simulink model "aeb"  (R2024a)
settings: Solver=VariableStepAuto  StartTime=0.0  StopTime=10.0  RelTol=1e-3
libraries: raspberrypisensorlib x1, autosarlibaprouting x1, raspberrypiNetworklib x1
settings Model: Creator=dahyun  LastModifiedBy=dahyun

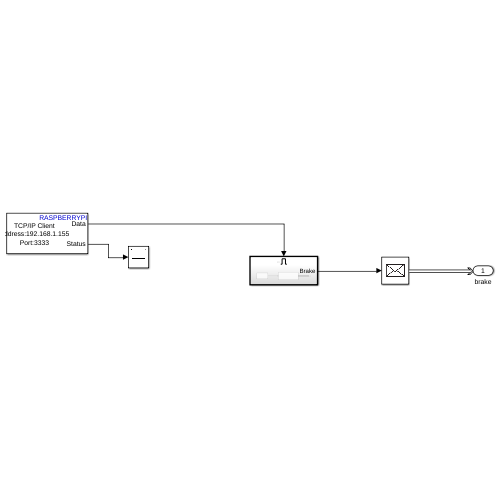
[thumbnail: Simulink's stored preview of the top-level diagram]
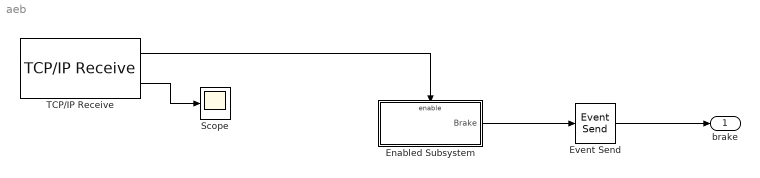
== system aeb ==
  Enabled Subsystem : Subsystem  TreatAsAtomicUnit=on
  Event Send : autosarlibaprouting/Event Send
  Scope : Scope
  TCP/IP Receive : raspberrypiNetworklib/TCP//IP Receive  Mode_=Client  LocalServerPort_=25000  RemoteAddr_=192.168.1.155  RemoteServerPort_=3333  DataType_=uint8  DataSize_=1  SampleTime_=0.1  SimulateUsing=Code generation  ClientPortBindingSelection_=off  ClientPortToBind_=35000  BlockingMode_=off  BlockTimeout_=0.1  BlockPlatform=RASPBERRYPI
  brake : Outport  InputPortMessageModes=m
  wires:
  Enabled Subsystem/1(Brake) -> Event Send/1
  TCP/IP Receive/2 -> Scope/1
  TCP/IP Receive/1 -> Enabled Subsystem/Enable
  Event Send/1 -> brake/1

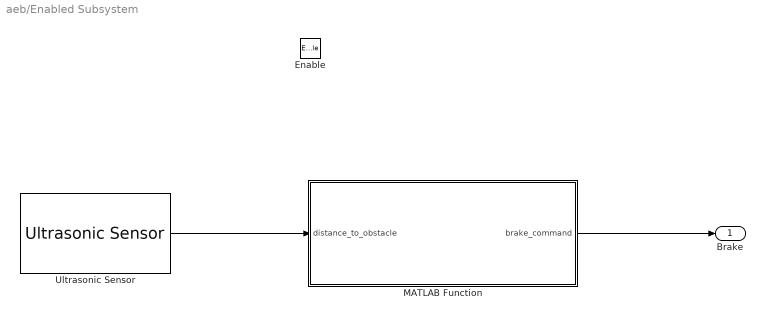
== system aeb/Enabled Subsystem ==
  Enable : EnablePort
  MATLAB Function : MATLAB Function  TreatAsAtomicUnit=on
  Ultrasonic Sensor : raspberrypisensorlib/Ultrasonic Sensor  BoardProperty=Pi 4 Model B  NumSignalPins=2  TrigPin=GPIO 4  EchoPin=GPIO 17  SignalPin=GPIO 23  SampleTime=-1  BlockPlatform=RASPBERRYPI
  Brake : Outport  InputPortMessageModes=m
  wires:
  Ultrasonic Sensor/1 -> MATLAB Function/1(distance_to_obstacle)
  MATLAB Function/1(brake_command) -> Brake/1

== matlab function aeb/Enabled Subsystem/MATLAB Function ==
  data: distance_to_obstacle input; brake_command output
function brake_command = aeb_system(distance_to_obstacle)
    % Define parameters
    threshold_distance = 0.12; % Threshold distance for AEB activation (in meters)
    % min_speed = 10; % Minimum vehicle speed for AEB activation (in m/s)

    % Check if AEB should activate based on distance and speed
    if distance_to_obstacle < threshold_distance
        brake_command = 1.0; % Activate brakes
    else
        brake_command = 0.0; % Do not activate brakes
    end
end
